simulink library "common_lib"  (Simulink 7.8)
settings: Solver=ode45  StartTime=0.0  StopTime=10.0  RelTol=1e-3
libraries: simulink x1
settings Model: Creator=fguerin  LastModifiedBy=fguerin

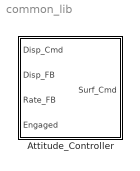
== system common_lib ==
  Attitude_Controller : Subsystem  mask(Attitude_Controller){dispGain=0, dispLim=0, rateGain=0, rateLim=0, intGain=0, intLim=0, cmdLim=0}
      mask prompts: dispLim "DispLimit (-/+)"; rateLim "RateLimit (+/-)"; intLim "IntLimit (+/-)"; cmdLim "CommandLimit (+/-)"
      mask help: This block performs attitude Control using displacement, rate and integral

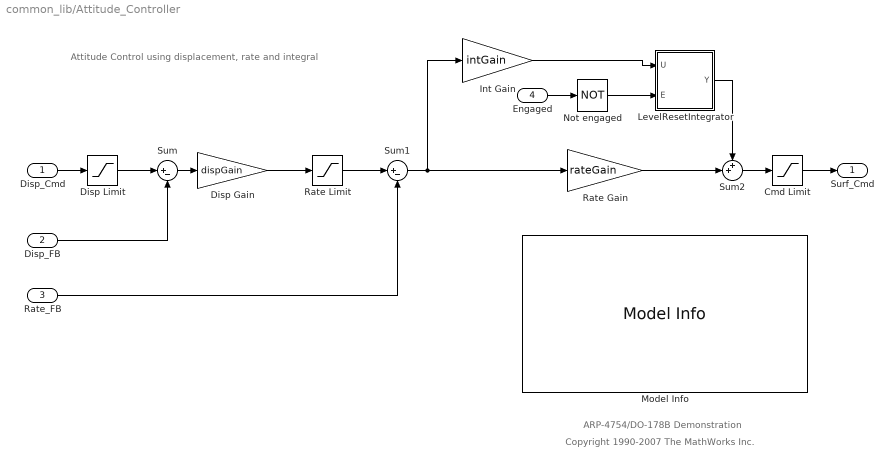
== system common_lib/Attitude_Controller ==
  note: Attitude Control using displacement, rate and integral
  note: Copyright 1990-2007 The MathWorks Inc.
  note: ARP-4754/DO-178B Demonstration
  Disp_Cmd : Inport  RequirementInfo={} %GIDa_208d03b8_4a6c_4cb5_8bcb_2be8ab486bbd  OutDataTypeStr=double  PortDimensions=1  SampleTime=1/40
  "Disp_FB " : Inport  RequirementInfo={} %GIDa_f3c5158a_8977_4be4_86c5_c87d37f9694b  Port=2  OutDataTypeStr=double  PortDimensions=1  SampleTime=1/40
  Rate_FB : Inport  RequirementInfo={} %GIDa_c36c3a16_e707_45e1_9087_e7fc8807fa47  Port=3  OutDataTypeStr=double  PortDimensions=1  SampleTime=1/40
  Engaged : Inport  RequirementInfo={} %GIDa_b77c6d1f_6f5c_4287_a539_b30ba18dd9c5  Port=4  OutDataTypeStr=boolean  PortDimensions=1  SampleTime=1/40
  Cmd Limit : Saturate  RequirementInfo={} %GIDa_5dbb5d06_d164_42c6_9c62_176d31276e7a  UpperLimit=cmdLim  LowerLimit=-cmdLim
      settings: AttributesFormatString=%<LowerLimit> to %<UpperLimit> (deg)
  Disp Gain : Gain  RequirementInfo={} %GIDa_9e97afa1_30fe_4be2_bc89_29b5921fc8c5  Gain=dispGain
  Disp Limit : Saturate  RequirementInfo={} %GIDa_9e660690_dca8_48ec_807d_b47291088128  UpperLimit=dispLim  LowerLimit=-dispLim
      settings: AttributesFormatString=%<LowerLimit> to %<UpperLimit> (deg)
  Int Gain : Gain  RequirementInfo={} %GIDa_870a0879_555c_4017_a3ba_c0edd2941a66  Gain=intGain
  LevelResetIntegrator : Subsystem  RequirementInfo={} %GIDa_01eaa2dd_251b_4e55_b9d4_77f00ed3c1e2  mask(SLCI_Level_Reset_Integrator){K=1.0, Ts=1/40, IC=0, UL=intLim, LL=-intLim}
      mask prompts: K "Gain value:"; Ts "Sample time (-1 for inherited):"; IC "Initial condition:"; UL "Upper saturation limit:"; LL "Lower saturation limit:"
      mask help: Level reset integrator using Forward Euler method. This masked subsystem implements the functional behavior of Simulink's Descrete-Time Integrator block using Simulink Code Inspector supported blocks.
      settings: AttributesFormatString=-%<LL> to %<UL>\n(deg)
      mask Display: fprintf('K Ts\n____\nz-1')
  Model Info : simulink/Model-Wide Utilities/Model Info  RequirementInfo={} %GIDa_f518c114_c190_4bcf_9e43_64bd1a3d47b9  InitialBlockCM=None  BlockCM=None  Frame=on  DisplayStringWithTags=|  HorizontalTextAlignment=Left  LeftAlignmentValue=0.02  SourceBlockDiagram=common_lib  TagMaxNumber=20
      | Attitude Controller
      | Author: %<LastModifiedBy>
      | Version: %<ModelVersion>
      | Date: %<LastModificationDate>
      | DO-178B Software Lifecycle Data:
      |   11.9 Software Requirements Data
      |   11.10 Design Description
      | DO-178B Objectives:
      |   5.2.1a Low Level Requirements are Developed
      |   5.2.1a Software Architecture is Developed
      |   5.2.1b  Derived Low Level Requirements are Developed
  Not engaged : Logic  RequirementInfo={} %GIDa_2b815307_6627_4e92_9aef_f80a8dd28bb3  Operator=NOT  IconShape=distinctive  AllPortsSameDT=off  OutDataTypeStr=boolean
  Rate Gain : Gain  RequirementInfo={} %GIDa_54d200e7_1113_4121_9617_82f0d541e01f  Gain=rateGain
  Rate Limit : Saturate  RequirementInfo={} %GIDa_3aac2272_defa_413c_a992_b9b339ae59c5  UpperLimit=rateLim  LowerLimit=-rateLim
      settings: AttributesFormatString=%<LowerLimit> to %<UpperLimit> (deg/sec)
  Sum : Sum  RequirementInfo={} %GIDa_b8f65d0c_e0e5_4ac7_8b4e_c6486b552eed  Inputs=|+-
  Sum1 : Sum  RequirementInfo={} %GIDa_a7ce8a48_2da4_4e14_b3db_a2622ddfde11  Inputs=|+-
  Sum2 : Sum  RequirementInfo={} %GIDa_7ae65fe5_b56d_4043_89cb_986fe471301b  Inputs=++|
  Surf_Cmd : Outport  RequirementInfo={} %GIDa_c647428d_90c2_435e_bdc4_2d471cd93dcd  OutDataTypeStr=double  PortDimensions=1  SampleTime=1/40
  wires:
  Disp_Cmd/1 -> Disp Limit/1
  "Disp_FB "/1 -> Sum/2
  Rate_FB/1 -> Sum1/2
  Sum1/1 -> Rate Gain/1, Int Gain/1
  Disp Gain/1 -> Rate Limit/1
  Sum/1 -> Disp Gain/1
  Disp Limit/1 -> Sum/1
  Rate Limit/1 -> Sum1/1
  Cmd Limit/1 -> Surf_Cmd/1
  Rate Gain/1 -> Sum2/2
  Sum2/1 -> Cmd Limit/1
  Engaged/1 -> Not engaged/1
  Not engaged/1 -> LevelResetIntegrator/2(E)
  LevelResetIntegrator/1(Y) -> Sum2/1
  Int Gain/1 -> LevelResetIntegrator/1(U)

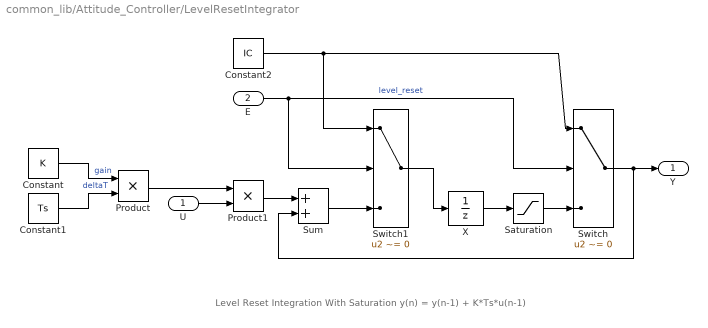
== system common_lib/Attitude_Controller/LevelResetIntegrator ==
  note: Level Reset Integration With Saturation
      | y(n) = y(n-1) + K*Ts*u(n-1)
  U : Inport
  E : Inport  Port=2
  Constant : Constant  Value=K
  Constant1 : Constant  Value=Ts
  Constant2 : Constant  Value=IC
  Product : Product  RndMeth=Zero
  Product1 : Product  RndMeth=Zero
  Saturation : Saturate  UpperLimit=UL  LowerLimit=LL
  Sum : Sum
  Switch : Switch  Criteria=u2 ~= 0
  Switch1 : Switch  Criteria=u2 ~= 0
  X : UnitDelay  X0=IC  SampleTime=Ts
  Y : Outport
  wires:
  Switch/1 -> Sum/2, Y/1
  Constant2/1 -> Switch/1, Switch1/1
  Saturation/1 -> Switch/3
  Product1/1 -> Sum/1
  X/1 -> Saturation/1
  U/1 -> Product1/2
  Product/1 -> Product1/1
  Constant1/1 -> Product/2  "deltaT"
  Constant/1 -> Product/1  "gain"
  Switch1/1 -> X/1
  Sum/1 -> Switch1/3
  E/1 -> Switch/2, Switch1/2  "level_reset"
